simulink model "Copter_Controller_discrete_sfun"  (Simulink 7.4)
settings: Solver=FixedStepDiscrete  StartTime=0.0  StopTime=tend  FixedStep=Ts  RelTol=1e-3
values from neighbouring files (symbols this model uses):
  g = 9.81    [complementary_filter_param.m]    (also in quadrocopter_param.m)
  m = elec.m+bat.m+boom.m+(4*mot.m)+(4*rot.m)    [quadrocopter_param.m]
  shift = 1000    [quadrocopter_param.m]
undefined symbols (not defined in the file or in its folder): despitch, desroll, desyaw
libraries: simulink x6
settings Model: Creator=Sreekanth  LastModifiedBy=Sreekanth
settings DataIOCC: LimitDataPoints=off
settings ConfigComp: Description=Design Verifier Custom Configuration Component  DVMaxProcessTime=600  DVDisplayUnsatisfiableObjectives=on  DVAutomaticStubbing=off  DVModelCoverageObjectives=MCDC  DVMaxTestCaseSteps=500  DVTestSuiteOptimization=CombinedObjectives  DVSaveHarnessModel=on  DVSaveReport=on

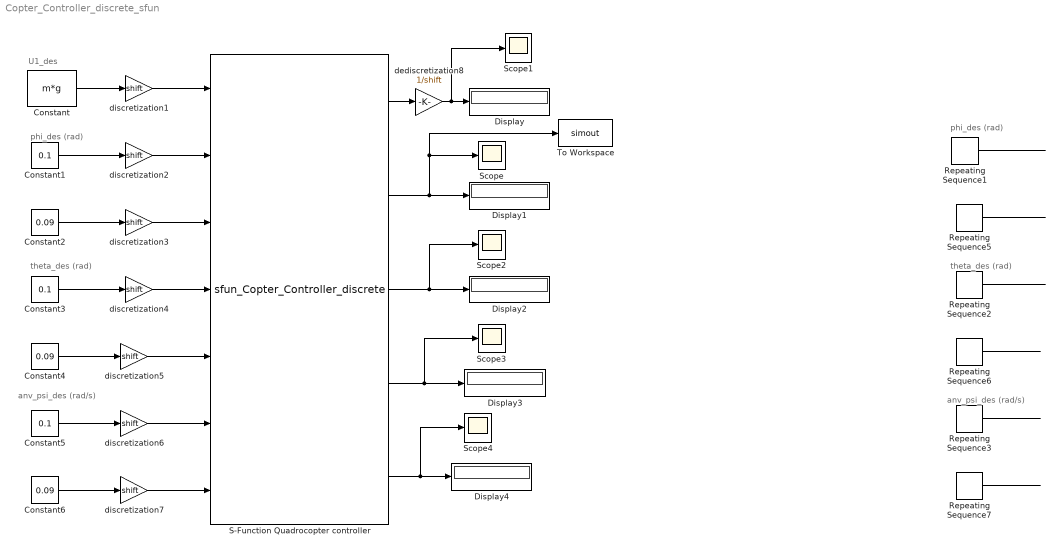
== system Copter_Controller_discrete_sfun ==
  note: U1_des
  note: phi_des (rad)
  note: theta_des (rad)
  note: anv_psi_des (rad/s)
  note: phi_des (rad)
  note: theta_des (rad)
  note: anv_psi_des (rad/s)
  Constant : Constant  Value=m*g  OutDataTypeMode=double  OutDataType=fixdt(1, 16)  OutScaling=2^0  OutDataTypeStr=double
  Constant1 : Constant  Value=0.1  OutDataType=fixdt(1, 16)  OutScaling=2^0
  Constant2 : Constant  Value=0.09  OutDataType=fixdt(1, 16)  OutScaling=2^0
  Constant3 : Constant  Value=0.1  OutDataType=fixdt(1, 16)  OutScaling=2^0
  Constant4 : Constant  Value=0.09  OutDataType=fixdt(1, 16)  OutScaling=2^0
  Constant5 : Constant  Value=0.1  OutDataType=fixdt(1, 16)  OutScaling=2^0
  Constant6 : Constant  Value=0.09  OutDataType=fixdt(1, 16)  OutScaling=2^0
  Display{,1..4} (5 alike) : Display
  Repeating Sequence1 : simulink/Sources/Repeating Sequence  SystemSampleTime=-1  rep_seq_t=desroll.time  rep_seq_y=desroll.angle
  Repeating Sequence2 : simulink/Sources/Repeating Sequence  SystemSampleTime=-1  rep_seq_t=despitch.time  rep_seq_y=despitch.angle
  Repeating Sequence3 : simulink/Sources/Repeating Sequence  SystemSampleTime=-1  rep_seq_t=desyaw.time  rep_seq_y=desyaw.velocity
  Repeating Sequence5 : simulink/Sources/Repeating Sequence  SystemSampleTime=-1  rep_seq_t=desroll.time  rep_seq_y=desroll.angle*0.9
  Repeating Sequence6 : simulink/Sources/Repeating Sequence  SystemSampleTime=-1  rep_seq_t=despitch.time  rep_seq_y=despitch.angle*0.9
  Repeating Sequence7 : simulink/Sources/Repeating Sequence  SystemSampleTime=-1  rep_seq_t=desyaw.time  rep_seq_y=desyaw.velocity*0.9
  S-Function Quadrocopter controller : S-Function  FunctionName=sfun_Copter_Controller_discrete  Parameters=[1 1 1 1 1 1 1 1 1]  EnableBusSupport=off
      mask Display:
      | port_label('input',1,'U1_des')
      | port_label('input',2,'phi_des')
      | port_label('input',3,'phi_filt')
      | port_label('input',4,'theta_des')
      | port_label('input',5,'theta_filt')
      | port_label('input',6,'anv_psi_des')
      | port_label('input',7,'anv_psi')
      | port_label('output',1,'U1_out')
      | port_label('output',2,'anv_prop1')
      | port_label('output',3,'anv_prop2')
      | port_label('output',4,'anv_prop3')
      | port_label('output',5,'anv_prop4')
  Scope{,1..4} (5 alike) : Scope
      Scope settings: TimeRange=30  YMin=0  YMax=6000
      Scope2 settings: SaveName=ScopeData2
      Scope3 settings: SaveName=ScopeData3
      Scope4 settings: SaveName=ScopeData4
  To Workspace : ToWorkspace  VariableName=simout  SampleTime=-1  SaveFormat=Structure
  dediscretization8 : Gain  Gain=1/shift  ParameterDataType=fixdt(1, 16)  ParameterScaling=2^0  OutDataTypeMode=double  OutDataType=fixdt(1, 16)  OutScaling=2^0  OutDataTypeStr=double
  discretization{1..7} (7 alike) : Gain  Gain=shift  ParameterDataType=fixdt(1, 16)  ParameterScaling=2^0  OutDataTypeMode=int16  OutDataType=fixdt(1, 16)  OutScaling=2^0  OutDataTypeStr=int16
  wires:
  S-Function Quadrocopter controller/1 -> dediscretization8/1
  S-Function Quadrocopter controller/2 -> Display1/1, Scope/1, To Workspace/1
  S-Function Quadrocopter controller/3 -> Display2/1, Scope2/1
  S-Function Quadrocopter controller/4 -> Display3/1, Scope3/1
  S-Function Quadrocopter controller/5 -> Display4/1, Scope4/1
  dediscretization8/1 -> Display/1, Scope1/1
  Constant/1 -> discretization1/1
  discretization1/1 -> S-Function Quadrocopter controller/1
  discretization2/1 -> S-Function Quadrocopter controller/2
  discretization3/1 -> S-Function Quadrocopter controller/3
  discretization4/1 -> S-Function Quadrocopter controller/4
  discretization5/1 -> S-Function Quadrocopter controller/5
  discretization6/1 -> S-Function Quadrocopter controller/6
  discretization7/1 -> S-Function Quadrocopter controller/7
  Repeating Sequence1/1 -> ?
  Repeating Sequence2/1 -> ?
  Repeating Sequence3/1 -> ?
  Repeating Sequence5/1 -> ?
  Repeating Sequence6/1 -> ?
  Repeating Sequence7/1 -> ?
  Constant2/1 -> discretization3/1
  Constant4/1 -> discretization5/1
  Constant6/1 -> discretization7/1
  Constant1/1 -> discretization2/1
  Constant3/1 -> discretization4/1
  Constant5/1 -> discretization6/1
